simulink model "Yaw_LQIDG"  (R2020a)
settings: Solver=ode3  StartTime=0.0  StopTime=10  FixedStep=0.02  RelTol=1e-3
InitFcn:
  | OpenLoop_LQDG_riccati_solver
values from neighbouring files (symbols this model uses):
  C3 = (m3 * g * miu_k * r_z) / (J_zz)    [QuadConstants.m]
  LQIDG_openloop_gain = (R1_inv * B' * p1)    [OpenLoop_LQDG_riccati_solver.m]
libraries: simulink x1, eeGeneralControl x1
settings Model: Creator=Ali  LastModifiedBy=Ali

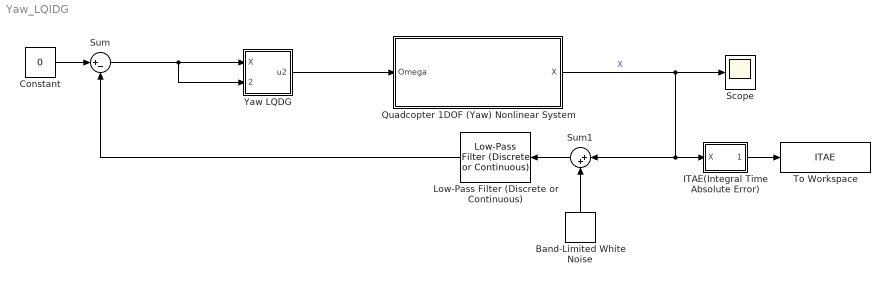
== system Yaw_LQIDG ==
  Band-Limited White Noise : simulink/Sources/Band-Limited White Noise  Cov=[0.0001]  Ts=0.02  seed=[23341]
  Constant : Constant  Value=0
  ITAE(Integral Time Absolute Error) : Subsystem
  Low-Pass Filter (Discrete or Continuous) : eeGeneralControl/Low-Pass Filter (Discrete or Continuous)  K=1  T=0.05  B=inf  A=-inf  init_option=Inherited from block input  x0=0  Ts=0
  Quadcopter 1DOF (Yaw) Nonlinear System : Subsystem  TreatAsAtomicUnit=on
      mask Display: image('quad1.png'); % Use "Edit Image" on toolstrip to change.
  Scope : Scope
  Sum : Sum  Inputs=|+-
  Sum1 : Sum  Inputs=|++
  To Workspace : ToWorkspace  VariableName=ITAE  SaveFormat=Timeseries  SampleTime=-1
  Yaw LQDG : Subsystem
  wires:
  Quadcopter 1DOF (Yaw) Nonlinear System/1(X) -> Sum1/1, ITAE(Integral Time Absolute Error)/1(X), Scope/1  "X"
  Constant/1 -> Sum/1
  ITAE(Integral Time Absolute Error)/1(ITAE) -> To Workspace/1
  Band-Limited White Noise/1 -> Sum1/2
  Sum1/1 -> Low-Pass Filter (Discrete or Continuous)/1
  Yaw LQDG/1(u2) -> Quadcopter 1DOF (Yaw) Nonlinear System/1(Omega)
  Sum/1 -> Yaw LQDG/2(Error), Yaw LQDG/1(X)
  Low-Pass Filter (Discrete or Continuous)/1 -> Sum/2

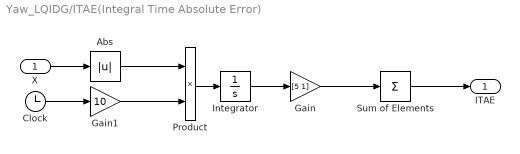
== system Yaw_LQIDG/ITAE(Integral Time Absolute Error) ==
  X : Inport
  Abs : Abs
  Clock : Clock
  Gain : Gain  Gain=[5 1]
  Gain1 : Gain  Gain=10
  Integrator : Integrator
  Product : Product
  Sum of Elements : Sum  Inputs=+
  ITAE : Outport
  wires:
  Product/1 -> Integrator/1
  Integrator/1 -> Gain/1
  Clock/1 -> Gain1/1
  Sum of Elements/1 -> ITAE/1
  Abs/1 -> Product/1
  X/1 -> Abs/1
  Gain/1 -> Sum of Elements/1
  Gain1/1 -> Product/2

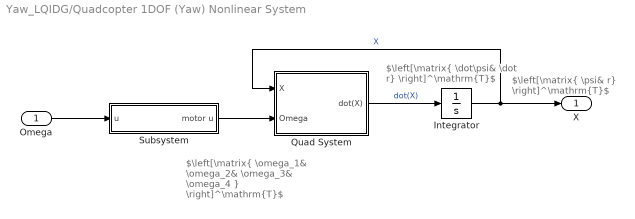
== system Yaw_LQIDG/Quadcopter 1DOF (Yaw) Nonlinear System ==
  note: $\left[\matrix{ \dot\psi& \dot r} \right]^\mathrm{T}$
  note: $\left[\matrix{ \omega_1& \omega_2& \omega_3& \omega_4 } \right]^\mathrm{T}$
  note: $\left[\matrix{ \psi& r} \right]^\mathrm{T}$
  Omega : Inport
  Integrator : Integrator  InitialCondition=[1.5, 0]
  Quad System : Subsystem
  Subsystem : Subsystem
  X : Outport
  wires:
  Integrator/1 -> Quad System/1(X), X/1  "X"
  Quad System/1(dot(X)) -> Integrator/1  "dot(X)"
  Omega/1 -> Subsystem/1(u)
  Subsystem/1(motor u) -> Quad System/2(Omega)

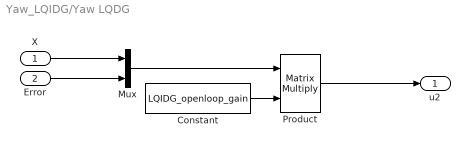
== system Yaw_LQIDG/Yaw LQDG ==
  X : Inport
  Error : Inport  Port=2
  Constant : Constant  Value=LQIDG_openloop_gain
  Mux : Mux  Inputs=2
  Product : Product  Multiplication=Matrix(*)
  u2 : Outport
  wires:
  Product/1 -> u2/1
  Constant/1 -> Product/2
  X/1 -> Mux/1
  Error/1 -> Mux/2
  Mux/1 -> Product/1

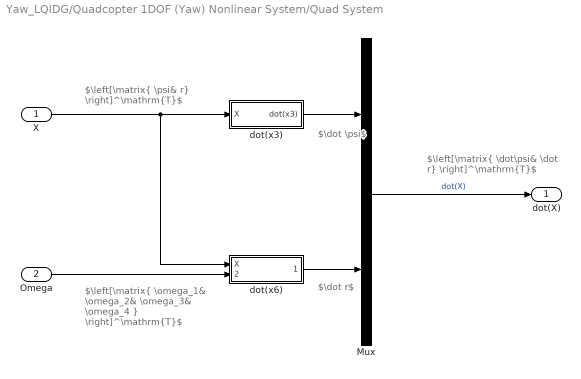
== system Yaw_LQIDG/Quadcopter 1DOF (Yaw) Nonlinear System/Quad System ==
  note: $\left[\matrix{ \omega_1& \omega_2& \omega_3& \omega_4 } \right]^\mathrm{T}$
  note: $\left[\matrix{ \dot\psi& \dot r} \right]^\mathrm{T}$
  note: $\dot \psi$
  note: $\dot r$
  note: $\left[\matrix{ \psi& r} \right]^\mathrm{T}$
  X : Inport
  Omega : Inport  Port=2
  Mux : Mux  Inputs=2
  dot(x3) : Subsystem
  dot(x6) : Subsystem
  dot(X) : Outport
  wires:
  Mux/1 -> dot(X)/1  "dot(X)"
  X/1 -> dot(x6)/1(X), dot(x3)/1(X)
  Omega/1 -> dot(x6)/2(Omega)
  dot(x3)/1(dot(x3)) -> Mux/1
  dot(x6)/1(dot(x6)) -> Mux/2

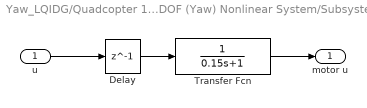
== system Yaw_LQIDG/Quadcopter 1DOF (Yaw) Nonlinear System/Subsystem ==
  u : Inport
  Delay : Delay  DelayLength=1
  Transfer Fcn : TransferFcn  Denominator=[0.15 1]
  motor u : Outport
  wires:
  Transfer Fcn/1 -> motor u/1
  u/1 -> Delay/1
  Delay/1 -> Transfer Fcn/1

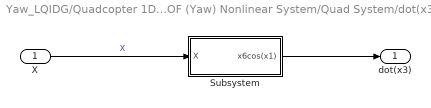
== system Yaw_LQIDG/Quadcopter 1DOF (Yaw) Nonlinear System/Quad System/dot(x3) ==
  X : Inport
  Subsystem : Subsystem
  dot(x3) : Outport
  wires:
  X/1 -> Subsystem/1(X)  "X"
  Subsystem/1(x6cos(x1)) -> dot(x3)/1

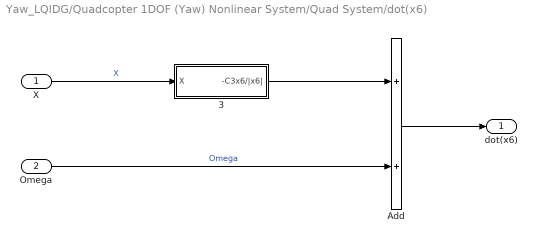
== system Yaw_LQIDG/Quadcopter 1DOF (Yaw) Nonlinear System/Quad System/dot(x6) ==
  X : Inport
  Omega : Inport  Port=2
  3 : Subsystem
  Add : Sum
  dot(x6) : Outport
  wires:
  Omega/1 -> Add/2  "Omega"
  Add/1 -> dot(x6)/1
  3/1("-C3x6/|x6| ") -> Add/1
  X/1 -> 3/1(X)  "X"

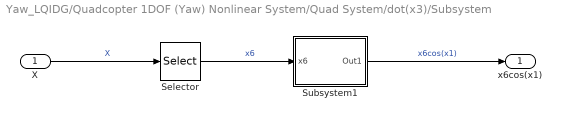
== system Yaw_LQIDG/Quadcopter 1DOF (Yaw) Nonlinear System/Quad System/dot(x3)/Subsystem ==
  X : Inport
  Selector : Selector  InputPortWidth=2  IndexOptions=Index vector (dialog)  Indices=[2]  OutputSizes=1
  Subsystem1 : Subsystem
  x6cos(x1) : Outport
  wires:
  Selector/1 -> Subsystem1/1(x6)  "x6"
  Subsystem1/1(Out1) -> x6cos(x1)/1  "x6cos(x1)"
  X/1 -> Selector/1  "X"

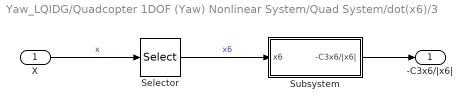
== system Yaw_LQIDG/Quadcopter 1DOF (Yaw) Nonlinear System/Quad System/dot(x6)/3 ==
  X : Inport
  Selector : Selector  InputPortWidth=2  IndexOptions=Index vector (dialog)  Indices=[2]  OutputSizes=1
  Subsystem : Subsystem
  "-C3x6/|x6| " : Outport
  wires:
  Selector/1 -> Subsystem/1(x6)  "x6"
  Subsystem/1("-C3x6/|x6| ") -> "-C3x6/|x6| "/1
  X/1 -> Selector/1  "x"

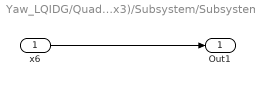
== system Yaw_LQIDG/Quadcopter 1DOF (Yaw) Nonlinear System/Quad System/dot(x3)/Subsystem/Subsystem1 ==
  x6 : Inport
  Out1 : Outport
  wires:
  x6/1 -> Out1/1

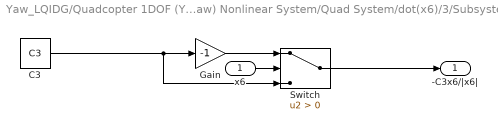
== system Yaw_LQIDG/Quadcopter 1DOF (Yaw) Nonlinear System/Quad System/dot(x6)/3/Subsystem ==
  x6 : Inport
  C3 : Constant  Value=C3
  Gain : Gain  Gain=-1
  Switch : Switch  Criteria=u2 > Threshold
  "-C3x6/|x6| " : Outport
  wires:
  Switch/1 -> "-C3x6/|x6| "/1
  C3/1 -> Switch/3, Gain/1
  x6/1 -> Switch/2
  Gain/1 -> Switch/1
